simulink model "SWC_STM"  (R2020a)
settings: Solver=FixedStepDiscrete  StartTime=0.0  StopTime=0.01  FixedStep=0.001  RelTol=1e-3
undefined symbols (not defined in the file or in its folder): CAL_STM_SpeedCtlMode_u8, CAL_STM_TrqSetRamp_f32, CAL_STM_UxptTrqLim_f32, CAL_STM_UxptTrqMonCountTrh_s16, CAL_STM_UxptTrqMonDebTrh_s16, CAL_STM_UxptTrqMonErrRst_b, GLB_STM_PosvTrq_u8, GLB_STM_ZeroTrq_u8
libraries: simulink x3
settings Model: DataDictionary=SWC_STM_DataDictionary.sldd  EnableAccessToBaseWorkspace=off  Creator=dongliyuan  LastModifiedBy=zhangjunren
settings DataIOCC: SaveFormat=StructureWithTime
settings OptimizationCC: DefaultParameterBehavior=Inlined  EnhancedBackFolding=on  PassReuseOutputArgsAs=Individual arguments  ZeroExternalMemoryAtStartup=off  ZeroInternalMemoryAtStartup=off  OptimizeBlockOrder=speed  DifferentSizesBufferReuse=on  OptimizationCustomize=off  EfficientTunableParamExpr=on
settings DebuggingCC: SignalInfNanChecking=warning  ParameterPrecisionLossMsg=none  ParameterTunabilityLossMsg=error  UnnecessaryDatatypeConvMsg=warning  VectorMatrixConversionMsg=warning  StrictBusMsg=WarnOnBusTreatedAsVector  NonBusSignalsTreatedAsBus=warning
settings ModelReferenceCC: ModelReferenceNumInstancesAllowed=Single
settings SFSimCC: MATLABDynamicMemAlloc=off
settings RTWCC: SystemTargetFile=ert.tlc  GenCodeOnly=on  TemplateMakefile=ert_default_tmf  CustomSourceCode="#include \"set_get_data.h\""
settings CodeAppCC: ForceParamTrailComments=on  IgnoreCustomStorageClasses=off  OperatorAnnotations=on  SimulinkDataObjDesc=on  SFDataObjDesc=on  InsertBlockDesc=on
settings ERTTargetCC: TargetLangStandard=C99 (ISO)  UtilityFuncGeneration=Shared location  IncludeMdlTerminateFcn=off  SupportNonFinite=off  SupportComplex=off  GenerateASAP2=on  InlinedParameterPlacement=NonHierarchical  ERTCustomFileTemplate=example_file_process.tlc  EnableUserReplacementTypes=on

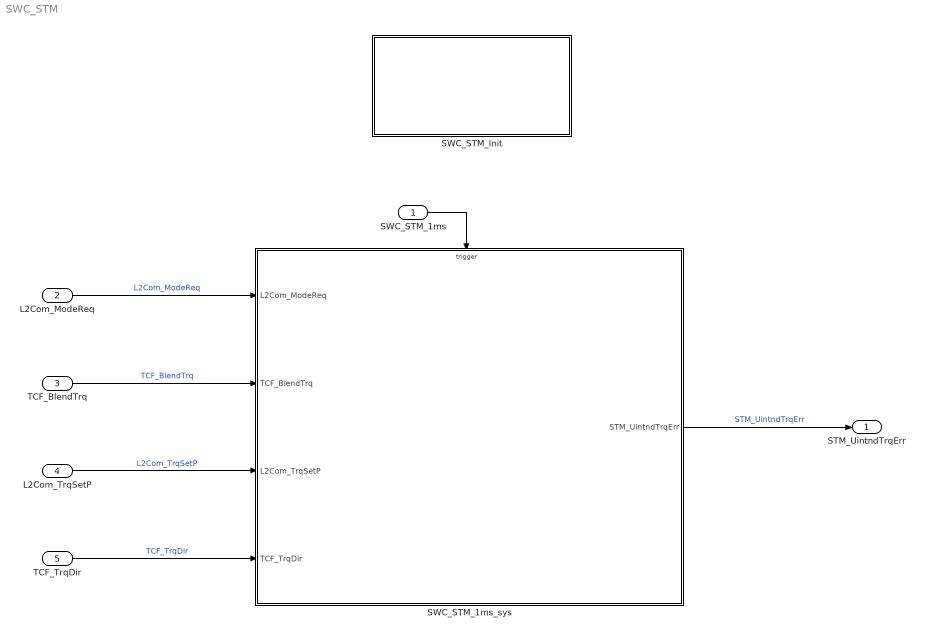
== system SWC_STM ==
  SWC_STM_1ms : Inport  SampleTime=0.001  OutputFunctionCall=on
  L2Com_ModeReq : Inport  Port=2  OutDataTypeStr=uint8  PortDimensions=1
  TCF_BlendTrq : Inport  Port=3  OutDataTypeStr=single  PortDimensions=1
  L2Com_TrqSetP : Inport  Port=4  OutDataTypeStr=single  PortDimensions=1
  TCF_TrqDir : Inport  Port=5  OutDataTypeStr=uint8  PortDimensions=1
  SWC_STM_1ms_sys : Subsystem
  SWC_STM_Init : Subsystem
  STM_UintndTrqErr : Outport
  wires:
  L2Com_TrqSetP/1 -> SWC_STM_1ms_sys/3(L2Com_TrqSetP)  "L2Com_TrqSetP"
  L2Com_ModeReq/1 -> SWC_STM_1ms_sys/1(L2Com_ModeReq)  "L2Com_ModeReq"
  SWC_STM_1ms/1 -> SWC_STM_1ms_sys/Trigger
  TCF_TrqDir/1 -> SWC_STM_1ms_sys/4(TCF_TrqDir)  "TCF_TrqDir"
  TCF_BlendTrq/1 -> SWC_STM_1ms_sys/2(TCF_BlendTrq)  "TCF_BlendTrq"
  SWC_STM_1ms_sys/1(STM_UintndTrqErr) -> STM_UintndTrqErr/1  "STM_UintndTrqErr"

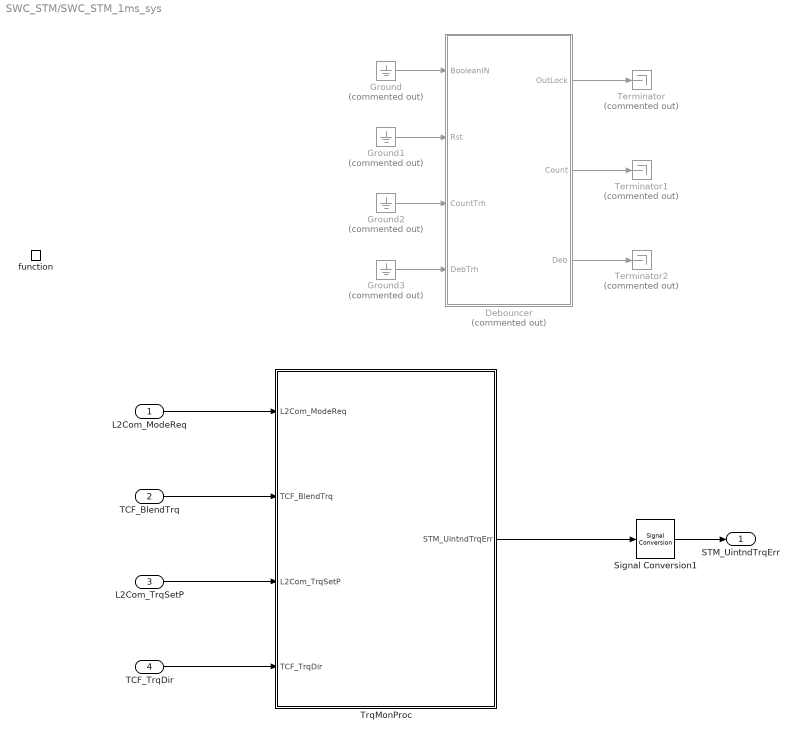
== system SWC_STM/SWC_STM_1ms_sys ==
  L2Com_ModeReq : Inport  OutDataTypeStr=uint8  PortDimensions=1
  TCF_BlendTrq : Inport  Port=2
  L2Com_TrqSetP : Inport  Port=3
  TCF_TrqDir : Inport  Port=4  OutDataTypeStr=uint8  PortDimensions=1
  function : TriggerPort  TriggerType=function-call  VariantControl=(inherit)  SampleTimeType=periodic  SampleTime=-1
  Debouncer : Subsystem  Commented=on  TreatAsAtomicUnit=on
  Ground{,1..3} (4 alike) : Ground  Commented=on
  Signal Conversion1 : SignalConversion  OverrideOpt=off
  Terminator : Terminator  Commented=on
  Terminator1 : Terminator  Commented=on
  Terminator2 : Terminator  Commented=on
  TrqMonProc : Subsystem
  STM_UintndTrqErr : Outport
  wires:
  Signal Conversion1/1 -> STM_UintndTrqErr/1
  TCF_BlendTrq/1 -> TrqMonProc/2(TCF_BlendTrq)
  L2Com_TrqSetP/1 -> TrqMonProc/3(L2Com_TrqSetP)
  TCF_TrqDir/1 -> TrqMonProc/4(TCF_TrqDir)
  TrqMonProc/1(STM_UintndTrqErr) -> Signal Conversion1/1
  L2Com_ModeReq/1 -> TrqMonProc/1(L2Com_ModeReq)
  Debouncer/1(OutLock) -> Terminator/1
  Debouncer/2(Count) -> Terminator1/1
  Debouncer/3(Deb) -> Terminator2/1
  Ground/1 -> Debouncer/1(BooleanIN)
  Ground1/1 -> Debouncer/2(Rst)
  Ground2/1 -> Debouncer/3(CountTrh)
  Ground3/1 -> Debouncer/4(DebTrh)

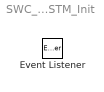
== system SWC_STM/SWC_STM_Init ==
  Event Listener : EventListener  EventName=reset

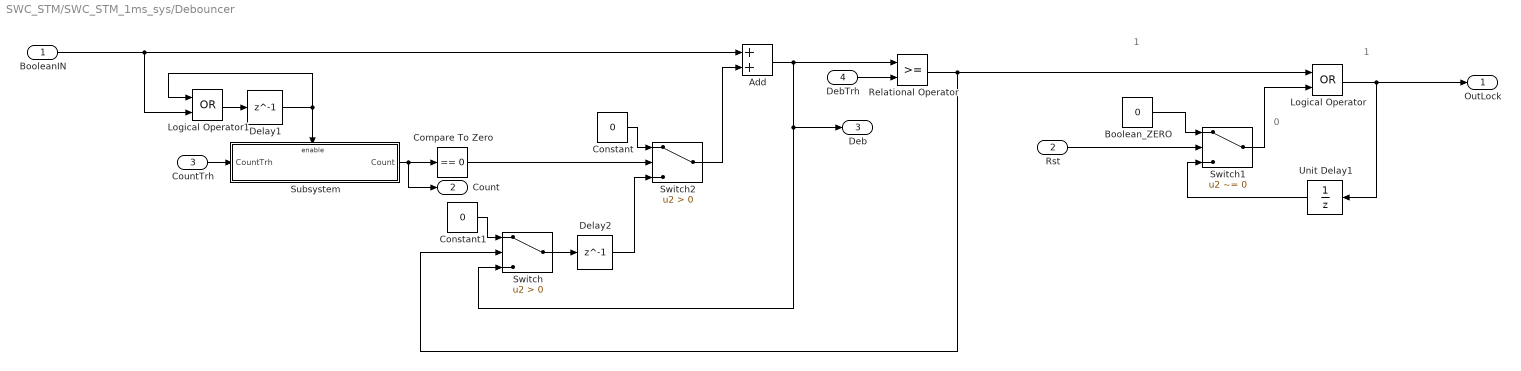
== system SWC_STM/SWC_STM_1ms_sys/Debouncer ==
  note: 0
  note: 1
  note: 1
  BooleanIN : Inport  OutDataTypeStr=boolean
  Rst : Inport  Port=2  OutDataTypeStr=boolean
  CountTrh : Inport  Port=3  OutDataTypeStr=int16
  DebTrh : Inport  Port=4  OutDataTypeStr=int16
  Add : Sum
  Boolean_ZERO : Constant  Value=0  OutDataTypeStr=boolean
  Compare To Zero : simulink/Logic and Bit Operations/Compare To Zero  relop===  OutDataTypeStr=boolean
  Constant : Constant  Value=0  OutDataTypeStr=int16
  Constant1 : Constant  Value=0  OutDataTypeStr=int16
  Delay1 : Delay  DelayLength=1
  Delay2 : Delay  DelayLength=1
  Logical Operator : Logic  Operator=OR  AllPortsSameDT=off  OutDataTypeStr=boolean
  Logical Operator1 : Logic  Operator=OR  AllPortsSameDT=off  OutDataTypeStr=boolean
  Relational Operator : RelationalOperator  OutDataTypeStr=boolean  RndMeth=Simplest
  Subsystem : Subsystem
  Switch : Switch  Criteria=u2 > Threshold
  Switch1 : Switch  Criteria=u2 ~= 0
  Switch2 : Switch  Criteria=u2 > Threshold
  Unit Delay1 : UnitDelay  SampleTime=-1  HasFrameUpgradeWarning=on
  OutLock : Outport  VectorParamsAs1DForOutWhenUnconnected=off
  Count : Outport  Port=2
  Deb : Outport  Port=3
  wires:
  Constant1/1 -> Switch/1
  Add/1 -> Relational Operator/1, Deb/1, Switch/3
  Switch/1 -> Delay2/1
  DebTrh/1 -> Relational Operator/2
  Relational Operator/1 -> Logical Operator/1, Switch/2
  BooleanIN/1 -> Add/1, Logical Operator1/2
  Unit Delay1/1 -> Switch1/3
  Switch1/1 -> Logical Operator/2
  Rst/1 -> Switch1/2
  Boolean_ZERO/1 -> Switch1/1
  Logical Operator/1 -> Unit Delay1/1, OutLock/1
  Subsystem/1(Count) -> Compare To Zero/1, Count/1
  Compare To Zero/1 -> Switch2/2
  Constant/1 -> Switch2/1
  Switch2/1 -> Add/2
  Delay1/1 -> Logical Operator1/1, Subsystem/Enable
  Logical Operator1/1 -> Delay1/1
  CountTrh/1 -> Subsystem/1(CountTrh)
  Delay2/1 -> Switch2/3

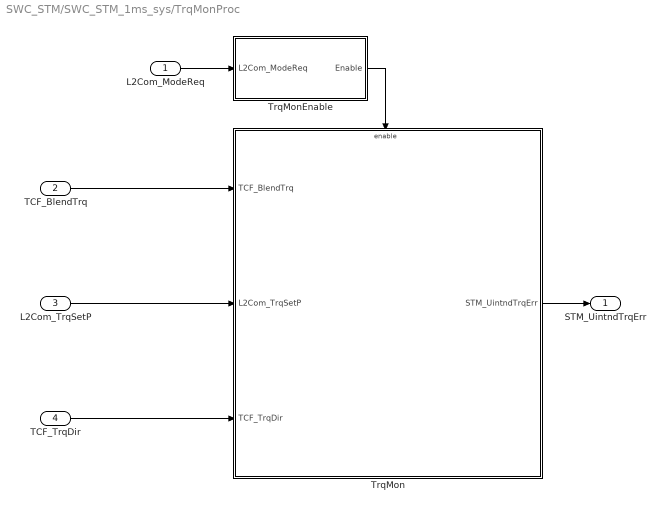
== system SWC_STM/SWC_STM_1ms_sys/TrqMonProc ==
  L2Com_ModeReq : Inport  OutDataTypeStr=uint8  PortDimensions=1
  TCF_BlendTrq : Inport  Port=2
  L2Com_TrqSetP : Inport  Port=3
  TCF_TrqDir : Inport  Port=4
  TrqMon : Subsystem
  TrqMonEnable : Subsystem  TreatAsAtomicUnit=on
  STM_UintndTrqErr : Outport
  wires:
  TCF_BlendTrq/1 -> TrqMon/1(TCF_BlendTrq)
  L2Com_TrqSetP/1 -> TrqMon/2(L2Com_TrqSetP)
  TCF_TrqDir/1 -> TrqMon/3(TCF_TrqDir)
  TrqMon/1(STM_UintndTrqErr) -> STM_UintndTrqErr/1
  L2Com_ModeReq/1 -> TrqMonEnable/1(L2Com_ModeReq)
  TrqMonEnable/1(Enable) -> TrqMon/Enable

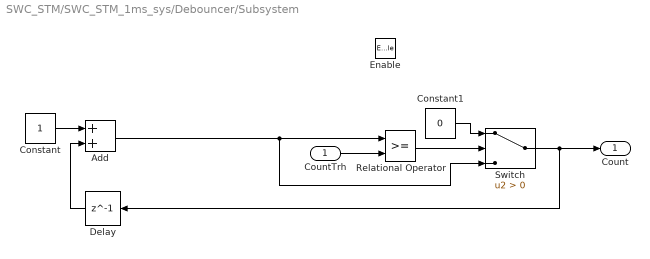
== system SWC_STM/SWC_STM_1ms_sys/Debouncer/Subsystem ==
  CountTrh : Inport
  Enable : EnablePort
  Add : Sum
  Constant : Constant  OutDataTypeStr=int16
  Constant1 : Constant  Value=0  OutDataTypeStr=int16
  Delay : Delay  DelayLength=1
  Relational Operator : RelationalOperator  OutDataTypeStr=boolean  RndMeth=Simplest
  Switch : Switch  Criteria=u2 > Threshold
  Count : Outport
  wires:
  Switch/1 -> Delay/1, Count/1
  Constant/1 -> Add/1
  Relational Operator/1 -> Switch/2
  Add/1 -> Relational Operator/1, Switch/3
  Constant1/1 -> Switch/1
  CountTrh/1 -> Relational Operator/2
  Delay/1 -> Add/2

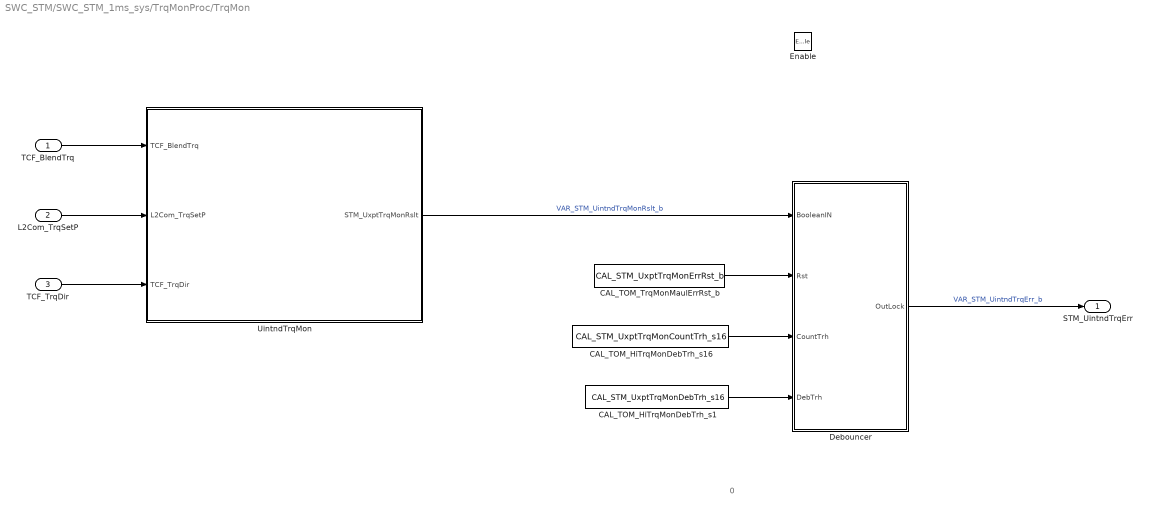
== system SWC_STM/SWC_STM_1ms_sys/TrqMonProc/TrqMon ==
  note: 0
  TCF_BlendTrq : Inport
  L2Com_TrqSetP : Inport  Port=2
  TCF_TrqDir : Inport  Port=3
  Enable : EnablePort
  CAL_TOM_HiTrqMonDebTrh_s1 : Constant  Value=CAL_STM_UxptTrqMonDebTrh_s16  OutDataTypeStr=int16
  CAL_TOM_HiTrqMonDebTrh_s16 : Constant  Value=CAL_STM_UxptTrqMonCountTrh_s16  OutDataTypeStr=int16
  CAL_TOM_TrqMonMaulErrRst_b : Constant  Value=CAL_STM_UxptTrqMonErrRst_b  OutDataTypeStr=boolean
  Debouncer : Subsystem  TreatAsAtomicUnit=on
  UintndTrqMon : Subsystem  TreatAsAtomicUnit=on
      settings: RTWSystemCode=Nonreusable function
  STM_UintndTrqErr : Outport
  wires:
  CAL_TOM_HiTrqMonDebTrh_s16/1 -> Debouncer/3(CountTrh)
  CAL_TOM_HiTrqMonDebTrh_s1/1 -> Debouncer/4(DebTrh)
  CAL_TOM_TrqMonMaulErrRst_b/1 -> Debouncer/2(Rst)
  TCF_BlendTrq/1 -> UintndTrqMon/1(TCF_BlendTrq)
  L2Com_TrqSetP/1 -> UintndTrqMon/2(L2Com_TrqSetP)
  TCF_TrqDir/1 -> UintndTrqMon/3(TCF_TrqDir)
  UintndTrqMon/1(STM_UxptTrqMonRslt) -> Debouncer/1(BooleanIN)  "VAR_STM_UintndTrqMonRslt_b"
  Debouncer/1(OutLock) -> STM_UintndTrqErr/1  "VAR_STM_UintndTrqErr_b"

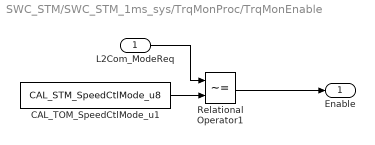
== system SWC_STM/SWC_STM_1ms_sys/TrqMonProc/TrqMonEnable ==
  L2Com_ModeReq : Inport  OutDataTypeStr=uint8  PortDimensions=1
  CAL_TOM_SpeedCtlMode_u1 : Constant  Value=CAL_STM_SpeedCtlMode_u8  OutDataTypeStr=uint8
  Relational Operator1 : RelationalOperator  Operator=~=  OutDataTypeStr=boolean  RndMeth=Simplest
  Enable : Outport
  wires:
  L2Com_ModeReq/1 -> Relational Operator1/1
  CAL_TOM_SpeedCtlMode_u1/1 -> Relational Operator1/2
  Relational Operator1/1 -> Enable/1

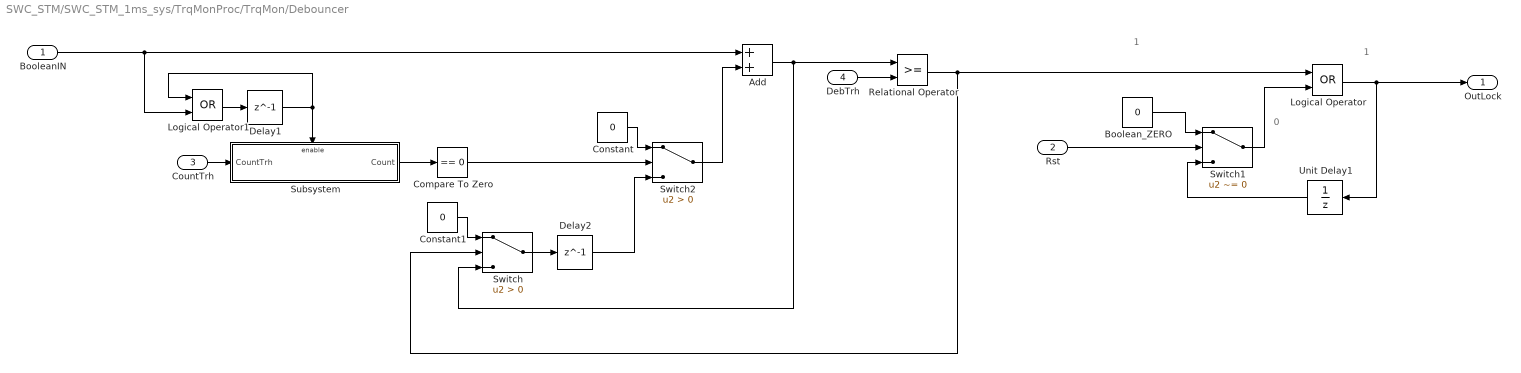
== system SWC_STM/SWC_STM_1ms_sys/TrqMonProc/TrqMon/Debouncer ==
  note: 0
  note: 1
  note: 1
  BooleanIN : Inport
  Rst : Inport  Port=2
  CountTrh : Inport  Port=3
  DebTrh : Inport  Port=4
  Add : Sum
  Boolean_ZERO : Constant  Value=0  OutDataTypeStr=boolean
  Compare To Zero : simulink/Logic and Bit Operations/Compare To Zero  relop===  OutDataTypeStr=boolean
  Constant : Constant  Value=0  OutDataTypeStr=int16
  Constant1 : Constant  Value=0  OutDataTypeStr=int16
  Delay1 : Delay  DelayLength=1
  Delay2 : Delay  DelayLength=1
  Logical Operator : Logic  Operator=OR  AllPortsSameDT=off  OutDataTypeStr=boolean
  Logical Operator1 : Logic  Operator=OR  AllPortsSameDT=off  OutDataTypeStr=boolean
  Relational Operator : RelationalOperator  OutDataTypeStr=boolean  RndMeth=Simplest
  Subsystem : Subsystem
  Switch : Switch  Criteria=u2 > Threshold
  Switch1 : Switch  Criteria=u2 ~= 0
  Switch2 : Switch  Criteria=u2 > Threshold
  Unit Delay1 : UnitDelay  SampleTime=-1  HasFrameUpgradeWarning=on
  OutLock : Outport  VectorParamsAs1DForOutWhenUnconnected=off
  wires:
  Constant1/1 -> Switch/1
  Add/1 -> Relational Operator/1, Switch/3
  Switch/1 -> Delay2/1
  DebTrh/1 -> Relational Operator/2
  Relational Operator/1 -> Logical Operator/1, Switch/2
  BooleanIN/1 -> Add/1, Logical Operator1/2
  Unit Delay1/1 -> Switch1/3
  Switch1/1 -> Logical Operator/2
  Rst/1 -> Switch1/2
  Boolean_ZERO/1 -> Switch1/1
  Logical Operator/1 -> Unit Delay1/1, OutLock/1
  Subsystem/1(Count) -> Compare To Zero/1
  Compare To Zero/1 -> Switch2/2
  Constant/1 -> Switch2/1
  Switch2/1 -> Add/2
  Delay1/1 -> Logical Operator1/1, Subsystem/Enable
  Logical Operator1/1 -> Delay1/1
  CountTrh/1 -> Subsystem/1(CountTrh)
  Delay2/1 -> Switch2/3

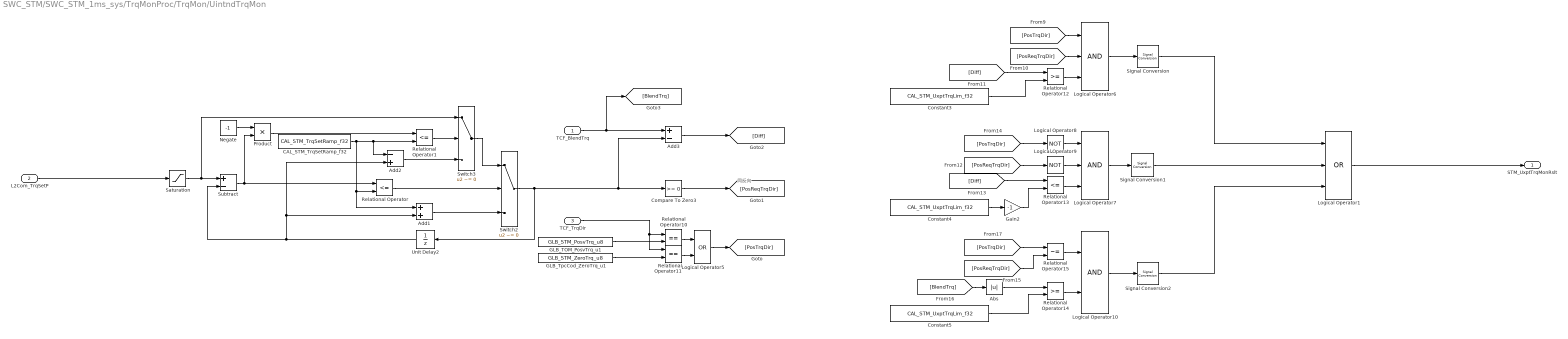
== system SWC_STM/SWC_STM_1ms_sys/TrqMonProc/TrqMon/UintndTrqMon ==
  note: 同反向
  TCF_BlendTrq : Inport
  L2Com_TrqSetP : Inport  Port=2
  TCF_TrqDir : Inport  Port=3
  Abs : Abs
  Add1 : Sum
  Add2 : Sum  Inputs=-+
  Add3 : Sum  Inputs=+-
  CAL_STM_TrqSetRamp_f32 : Constant  Value=CAL_STM_TrqSetRamp_f32
  Compare To Zero3 : simulink/Logic and Bit Operations/Compare To Zero  relop=>=  OutDataTypeStr=boolean
  Constant3 : Constant  Value=CAL_STM_UxptTrqLim_f32
  Constant4 : Constant  Value=CAL_STM_UxptTrqLim_f32
  Constant5 : Constant  Value=CAL_STM_UxptTrqLim_f32
  GLB_TOM_PosvTrq_u1 : Constant  Value=GLB_STM_PosvTrq_u8
  GLB_TpcCod_ZeroTrq_u1 : Constant  Value=GLB_STM_ZeroTrq_u8
  Gain2 : Gain  Gain=-1
  Logical Operator1 : Logic  Operator=OR  Inputs=3  AllPortsSameDT=off  OutDataTypeStr=boolean
  Logical Operator10 : Logic  AllPortsSameDT=off  OutDataTypeStr=boolean
  Logical Operator5 : Logic  Operator=OR  AllPortsSameDT=off  OutDataTypeStr=boolean
  Logical Operator6 : Logic  Inputs=3  AllPortsSameDT=off  OutDataTypeStr=boolean
  Logical Operator7 : Logic  Inputs=3  AllPortsSameDT=off  OutDataTypeStr=boolean
  Logical Operator8 : Logic  Operator=NOT  AllPortsSameDT=off  OutDataTypeStr=boolean
  Logical Operator9 : Logic  Operator=NOT  AllPortsSameDT=off  OutDataTypeStr=boolean
  Negate : Constant  Value=-1  OutDataTypeStr=single
  Product : Product
  Relational Operator : RelationalOperator  Operator=<=  OutDataTypeStr=boolean  RndMeth=Simplest
  Relational Operator1 : RelationalOperator  Operator=<=  OutDataTypeStr=boolean  RndMeth=Simplest
  Relational Operator10 : RelationalOperator  Operator===  OutDataTypeStr=boolean  RndMeth=Simplest
  Relational Operator11 : RelationalOperator  Operator===  OutDataTypeStr=boolean  RndMeth=Simplest
  Relational Operator12 : RelationalOperator  OutDataTypeStr=boolean  RndMeth=Simplest
  Relational Operator13 : RelationalOperator  Operator=<=  OutDataTypeStr=boolean  RndMeth=Simplest
  Relational Operator14 : RelationalOperator  OutDataTypeStr=boolean  RndMeth=Simplest
  Relational Operator15 : RelationalOperator  Operator=~=  OutDataTypeStr=boolean  RndMeth=Simplest
  Saturation : Saturate  UpperLimit=500  LowerLimit=-500
  Signal Conversion : SignalConversion  OverrideOpt=off
  Signal Conversion1 : SignalConversion  OverrideOpt=off
  Signal Conversion2 : SignalConversion  OverrideOpt=off
  Subtract : Sum  Inputs=+-
  Switch2 : Switch  Criteria=u2 ~= 0
  Switch3 : Switch  Criteria=u2 ~= 0
  Unit Delay2 : UnitDelay  SampleTime=-1  HasFrameUpgradeWarning=on
  STM_UxptTrqMonRslt : Outport
  wires:
  Relational Operator12/1 -> Logical Operator6/3
  [PosTrqDir] -> Logical Operator6/1
  Relational Operator15/1 -> Logical Operator10/1
  TCF_BlendTrq/1 -> [BlendTrq], Add3/1
  Constant3/1 -> Relational Operator12/2
  Relational Operator13/1 -> Logical Operator7/3
  Constant5/1 -> Relational Operator14/2
  Relational Operator11/1 -> Logical Operator5/2
  [BlendTrq] -> Abs/1
  Relational Operator10/1 -> Logical Operator5/1
  [Diff] -> Relational Operator12/1
  Logical Operator6/1 -> Signal Conversion/1
  TCF_TrqDir/1 -> Relational Operator10/1, Relational Operator11/1
  Logical Operator9/1 -> Logical Operator7/2
  GLB_TpcCod_ZeroTrq_u1/1 -> Relational Operator11/2
  [PosReqTrqDir] -> Relational Operator15/2
  Gain2/1 -> Relational Operator13/2
  Compare To Zero3/1 -> [PosReqTrqDir]
  Logical Operator8/1 -> Logical Operator7/1
  Logical Operator5/1 -> [PosTrqDir]
  Logical Operator10/1 -> Signal Conversion2/1
  [PosTrqDir] -> Relational Operator15/1
  GLB_TOM_PosvTrq_u1/1 -> Relational Operator10/2
  [Diff] -> Relational Operator13/1
  Relational Operator14/1 -> Logical Operator10/2
  Add3/1 -> [Diff]
  [PosReqTrqDir] -> Logical Operator6/2
  [PosReqTrqDir] -> Logical Operator9/1
  Logical Operator7/1 -> Signal Conversion1/1
  [PosTrqDir] -> Logical Operator8/1
  Abs/1 -> Relational Operator14/1
  Logical Operator1/1 -> STM_UxptTrqMonRslt/1
  Constant4/1 -> Gain2/1
  Signal Conversion/1 -> Logical Operator1/1
  Signal Conversion1/1 -> Logical Operator1/2
  Signal Conversion2/1 -> Logical Operator1/3
  Switch2/1 -> Add3/2, Compare To Zero3/1, Unit Delay2/1
  Negate/1 -> Product/1
  Switch3/1 -> Switch2/1
  Saturation/1 -> Switch3/1, Subtract/1
  Add2/1 -> Switch3/3
  CAL_STM_TrqSetRamp_f32/1 -> Add2/1, Relational Operator1/2, Relational Operator/2, Add1/1
  L2Com_TrqSetP/1 -> Saturation/1
  Subtract/1 -> Product/2, Relational Operator/1
  Add1/1 -> Switch2/3
  Unit Delay2/1 -> Subtract/2, Add1/2, Add2/2
  Relational Operator/1 -> Switch2/2
  Relational Operator1/1 -> Switch3/2
  Product/1 -> Relational Operator1/1

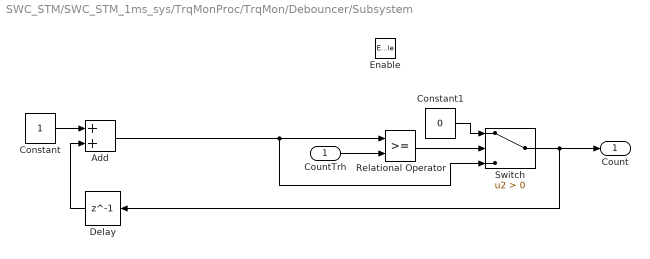
== system SWC_STM/SWC_STM_1ms_sys/TrqMonProc/TrqMon/Debouncer/Subsystem ==
  CountTrh : Inport
  Enable : EnablePort
  Add : Sum
  Constant : Constant  OutDataTypeStr=int16
  Constant1 : Constant  Value=0  OutDataTypeStr=int16
  Delay : Delay  DelayLength=1
  Relational Operator : RelationalOperator  OutDataTypeStr=boolean  RndMeth=Simplest
  Switch : Switch  Criteria=u2 > Threshold
  Count : Outport
  wires:
  Switch/1 -> Delay/1, Count/1
  Constant/1 -> Add/1
  Relational Operator/1 -> Switch/2
  Add/1 -> Relational Operator/1, Switch/3
  Constant1/1 -> Switch/1
  CountTrh/1 -> Relational Operator/2
  Delay/1 -> Add/2
